simulink model "saturate"  (Simulink 7.3)
settings: Solver=FixedStepDiscrete  StartTime=0.0  StopTime=10.0  FixedStep=1  RelTol=1e-3
settings Model: Creator=ksmyth  LastModifiedBy=hnine
settings OptimizationCC: InitFltsAndDblsToZero=on
settings DebuggingCC: SaveWithParameterizedLinksMsg=none
settings GRTTargetCC: TargetFcnLib=ansi_tfl_tmw.mat

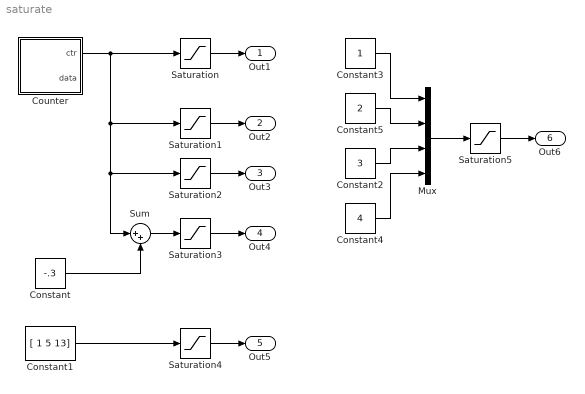
== system saturate ==
  Constant : Constant  Value=-.3  OutDataType=sfix(16)  OutScaling=2^0
  Constant1 : Constant  Value=[ 1 5 13]  OutDataType=sfix(16)  OutScaling=2^0
  Constant2 : Constant  Value=3  OutDataType=sfix(16)  OutScaling=2^0
  Constant3 : Constant  OutDataType=sfix(16)  OutScaling=2^0
  Constant4 : Constant  Value=4  OutDataType=sfix(16)  OutScaling=2^0
  Constant5 : Constant  Value=2  OutDataType=sfix(16)  OutScaling=2^0
  Counter : Stateflow chart
  Mux : Mux
  Saturation : Saturate  UpperLimit=2.3  LowerLimit=0.9
  Saturation1 : Saturate  UpperLimit=4  LowerLimit=1
  Saturation2 : Saturate  UpperLimit=4  LowerLimit=4
  Saturation3 : Saturate  UpperLimit=3  LowerLimit=1
  Saturation4 : Saturate  UpperLimit=[ 5 6 15]  LowerLimit=[ 3 5 10]
  Saturation5 : Saturate  UpperLimit=[ 3.5 3.5 3.5 inf ]  LowerLimit=[ 1.5 1.5 1.5 -inf ]  OutDataTypeStr=Inherit: Inherit via back propagation
  Sum : Sum  Inputs=|++  OutDataType=sfix(16)  OutScaling=2^0
  Out1 : Outport  OutDataType=sfix(16)  OutScaling=2^0
  Out2 : Outport  Port=2  OutDataType=sfix(16)  OutScaling=2^0
  Out3 : Outport  Port=3  OutDataType=sfix(16)  OutScaling=2^0
  Out4 : Outport  Port=4  OutDataType=sfix(16)  OutScaling=2^0
  Out5 : Outport  Port=5  OutDataType=sfix(16)  OutScaling=2^0
  Out6 : Outport  Port=6  PortDimensions=4  DataType=double  OutDataType=sfix(16)  OutScaling=2^0  OutDataTypeStr=double
  wires:
  Counter/1(ctr) -> Saturation/1, Saturation1/1, Saturation2/1, Sum/1
  Saturation/1 -> Out1/1
  Saturation1/1 -> Out2/1
  Saturation2/1 -> Out3/1
  Constant/1 -> Sum/2
  Sum/1 -> Saturation3/1
  Saturation3/1 -> Out4/1
  Saturation4/1 -> Out5/1
  Constant1/1 -> Saturation4/1
  Constant3/1 -> Mux/1
  Constant5/1 -> Mux/2
  Constant2/1 -> Mux/3
  Constant4/1 -> Mux/4
  Mux/1 -> Saturation5/1
  Saturation5/1 -> Out6/1

== stateflow chart Counter ==
  settings: executeAtInitialization=1
  state s1
  (default) -> s1
  s1 -> s1 [order 1] : [ctr < 4] / ctr = ctr+1;
  s1 -> s1 [order 2] : [ctr >= 4] / ctr = 0;
  data: ctr output double =1; data output double =-1
